simulink model "ASDdc_Governor"  (R2016b)
settings: configuration reference "CodeGenConfigSet" (kept outside this file)
values from neighbouring files (symbols this model uses):
  ASDdc_trqLimMax_C = Calibration.Parameter    [init_ASDdc_Governor.m]    (also in init_ASDdc_Governor_SIL.m = Simulink.Parameter)
  ASDdc_trqLimMin_C = Calibration.Parameter    [init_ASDdc_Governor.m]    (also in init_ASDdc_Governor_SIL.m = Simulink.Parameter)
  ASDdc_vLimIni_C = Calibration.Parameter    [init_ASDdc_Governor.m]    (also in init_ASDdc_Governor_SIL.m = Simulink.Parameter)
  PthSet_trqASDdcInit_C = Calibration.Parameter    [init_ASDdc_Governor.m]    (also in init_ASDdc_Governor_SIL.m = Simulink.Parameter)
undefined symbols (not defined in the file or in its folder): ASDdc_Governor_DT, EngState_conv
libraries: CXLib x3
settings Model: Creator=lenovo  LastModifiedBy=lenovo
settings ConfigSetRef: SourceLocation=Base Workspace

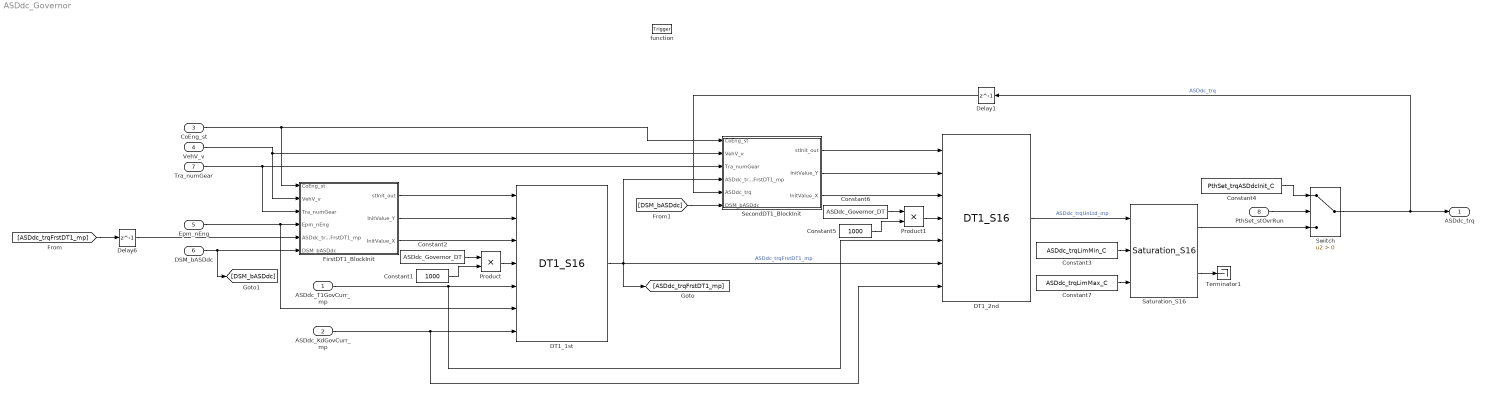
== system ASDdc_Governor ==
  ASDdc_T1GovCurr_mp : Inport  Tag=ms  Description=Current parameter T1 for ASD disturbance compensator  OutMin=0  OutMax=65535  OutDataTypeStr=RailDT1_ms
  ASDdc_KdGovCurr_mp : Inport  Description=Current parameter Kd for ASD disturbance compensator  Port=2  OutMin=0  OutMax=15  OutDataTypeStr=Pid_Kp_Kd
  CoEng_st : Inport  Description=Engine coordinator state  Port=3  OutDataTypeStr=Enum: EngState_conv
  VehV_v : Inport  Tag=km/h  Description=Vehicle speed  Port=4  OutMin=0  OutMax=250  OutDataTypeStr=VehSpeed_km_h
  Epm_nEng : Inport  Tag=rpm  Description=Engine speed  Port=5  OutMin=0  OutMax=6000  OutDataTypeStr=EngSpeed_rpm
  DSM_bASDdc : Inport  Description=state of Fid_ASDDc  Port=6  OutMin=0  OutMax=1  OutDataTypeStr=boolean
  Tra_numGear : Inport  Description=Current gear information  Port=7  OutMin=-128  OutMax=127  OutDataTypeStr=Tra_num
  PthSet_stOvrRun : Inport  Description=State of overrun detection (0: No overrun; 1: overrun)  Port=8  OutMin=0  OutMax=1  OutDataTypeStr=boolean
  function : TriggerPort  TriggerType=function-call  VariantControl=Variant
  Constant1 : Constant  RequirementInfo={'other' 'APP_requirements.doc' '@Simulink_requirement_item_25' 'true' '手动开关' '' } %GIDa_e3d2db55_e091_4804_b405_e3bf1d89a990  Value=1000  OutDataTypeStr=uint32
  Constant2 : Constant  RequirementInfo={'other' 'APP_requirements.doc' '@Simulink_requirement_item_25' 'true' '手动开关' '' } %GIDa_d3ebbc02_8a2a_474e_954c_97ec141fe6cb  Value=ASDdc_Governor_DT
  Constant3 : Constant  RequirementInfo={'other' 'APP_requirements.doc' '@Simulink_requirement_item_25' 'true' '手动开关' '' } %GIDa_af684717_0e96_4c26_8bce_fac0e3667dc0  Value=ASDdc_trqLimMin_C  SampleTime=-1
  Constant4 : Constant  RequirementInfo={'other' 'APP_requirements.doc' '@Simulink_requirement_item_25' 'true' '手动开关' '' } %GIDa_d8318f6c_a07c_4d1c_adda_9fb670b3e1e3  Value=PthSet_trqASDdcInit_C  SampleTime=-1
  Constant5 : Constant  RequirementInfo={'other' 'APP_requirements.doc' '@Simulink_requirement_item_25' 'true' '手动开关' '' } %GIDa_6b95edb5_017f_4d36_805f_c1c3801a481a  Value=1000  OutDataTypeStr=uint32
  Constant6 : Constant  RequirementInfo={'other' 'APP_requirements.doc' '@Simulink_requirement_item_25' 'true' '手动开关' '' } %GIDa_682dba5f_241e_4249_aa6e_798392b0670d  Value=ASDdc_Governor_DT
  Constant7 : Constant  RequirementInfo={'other' 'APP_requirements.doc' '@Simulink_requirement_item_25' 'true' '手动开关' '' } %GIDa_b9d68d89_a686_4446_af65_722001efe125  Value=ASDdc_trqLimMax_C  SampleTime=-1
  DT1_1st : CXLib/DT1_S16
  DT1_2nd : CXLib/DT1_S16
  Delay1 : Delay  DelayLength=1  InitialCondition=0
  Delay6 : Delay  DelayLength=1  InitialCondition=0
  FirstDT1_BlockInit : Subsystem
  Product : Product  OutDataTypeStr=Inherit: Inherit via back propagation
  Product1 : Product  OutDataTypeStr=Inherit: Inherit via back propagation
  Saturation_S16 : CXLib/Saturation_S16
  SecondDT1_BlockInit : Subsystem
  Switch : Switch  Criteria=u2 > Threshold
  Terminator1 : Terminator
  ASDdc_trq : Outport  Tag=Nm  Description=ASD disturbance compensator torque output  OutMin=-3000  OutMax=3000  OutDataTypeStr=Trq_Nm
  wires:
  Delay1/1 -> SecondDT1_BlockInit/5(ASDdc_trq)
  Delay6/1 -> FirstDT1_BlockInit/5(ASDdc_trqFrstDT1_mp)
  [ASDdc_trqFrstDT1_mp] -> Delay6/1
  Tra_numGear/1 -> FirstDT1_BlockInit/3(Tra_numGear), SecondDT1_BlockInit/3(Tra_numGear)
  Epm_nEng/1 -> DT1_1st/6, FirstDT1_BlockInit/4(Epm_nEng)
  SecondDT1_BlockInit/1(stInit_out) -> DT1_2nd/1
  SecondDT1_BlockInit/2(InitValue_Y) -> DT1_2nd/2
  SecondDT1_BlockInit/3(InitValue_X) -> DT1_2nd/3
  FirstDT1_BlockInit/1(stInit_out) -> DT1_1st/1
  FirstDT1_BlockInit/2(InitValue_Y) -> DT1_1st/2
  FirstDT1_BlockInit/3(InitValue_X) -> DT1_1st/3
  ASDdc_KdGovCurr_mp/1 -> DT1_2nd/7, DT1_1st/7
  ASDdc_T1GovCurr_mp/1 -> DT1_2nd/5, DT1_1st/5
  VehV_v/1 -> FirstDT1_BlockInit/2(VehV_v), SecondDT1_BlockInit/2(VehV_v)
  CoEng_st/1 -> FirstDT1_BlockInit/1(CoEng_st), SecondDT1_BlockInit/1(CoEng_st)
  Switch/1 -> ASDdc_trq/1, Delay1/1  "ASDdc_trq"
  Saturation_S16/2 -> Terminator1/1
  Constant7/1 -> Saturation_S16/3
  Constant3/1 -> Saturation_S16/2
  DT1_2nd/1 -> Saturation_S16/1  "ASDdc_trqUnLtd_mp"
  DT1_1st/1 -> SecondDT1_BlockInit/4(ASDdc_trqFrstDT1_mp), DT1_2nd/6, [ASDdc_trqFrstDT1_mp]  "ASDdc_trqFrstDT1_mp"
  DSM_bASDdc/1 -> FirstDT1_BlockInit/6(DSM_bASDdc), [DSM_bASDdc]
  [DSM_bASDdc] -> SecondDT1_BlockInit/6(DSM_bASDdc)
  Product/1 -> DT1_1st/4
  Constant2/1 -> Product/1
  Constant1/1 -> Product/2
  Constant6/1 -> Product1/1
  Constant5/1 -> Product1/2
  Product1/1 -> DT1_2nd/4
  PthSet_stOvrRun/1 -> Switch/2
  Saturation_S16/1 -> Switch/3
  Constant4/1 -> Switch/1

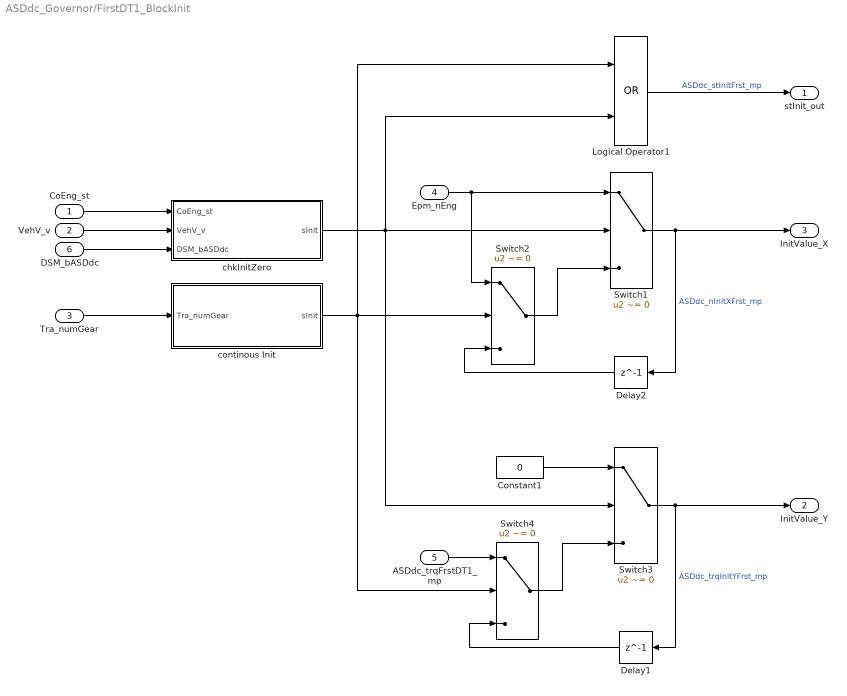
== system ASDdc_Governor/FirstDT1_BlockInit ==
  CoEng_st : Inport
  VehV_v : Inport  Port=2
  Tra_numGear : Inport  Port=3
  Epm_nEng : Inport  Port=4
  ASDdc_trqFrstDT1_mp : Inport  Port=5
  DSM_bASDdc : Inport  Description=state of Fid_ASDDc  Port=6
  Constant1 : Constant  RequirementInfo={'other' 'APP_requirements.doc' '@Simulink_requirement_item_25' 'true' '手动开关' '' } %GIDa_41ce0f65_227c_46f1_80d2_1d565a574450  Value=0  OutDataTypeStr=Inherit: Inherit via back propagation
  Delay1 : Delay  DelayLength=1  InitialCondition=0
  Delay2 : Delay  DelayLength=1  InitialCondition=0
  Logical Operator1 : Logic  Operator=OR  OutDataTypeStr=boolean
  Switch{1..4} (4 alike) : Switch  Criteria=u2 ~= 0  SaturateOnIntegerOverflow=on  InputSameDT=on
  chkInitZero : Subsystem
  continous Init : Subsystem
  stInit_out : Outport
  InitValue_Y : Outport  Port=2
  InitValue_X : Outport  Port=3
  wires:
  Tra_numGear/1 -> continous Init/1(Tra_numGear)
  VehV_v/1 -> chkInitZero/2(VehV_v)
  CoEng_st/1 -> chkInitZero/1(CoEng_st)
  ASDdc_trqFrstDT1_mp/1 -> Switch4/1
  Epm_nEng/1 -> Switch1/1, Switch2/1
  continous Init/1(sInit) -> Logical Operator1/1, Switch2/2, Switch4/2
  Switch3/1 -> Delay1/1, InitValue_Y/1  "ASDdc_trqInitYFrst_mp"
  Constant1/1 -> Switch3/1
  chkInitZero/1(sInit) -> Logical Operator1/2, Switch1/2, Switch3/2
  Switch4/1 -> Switch3/3
  Delay1/1 -> Switch4/3
  Logical Operator1/1 -> stInit_out/1  "ASDdc_stInitFrst_mp"
  Switch2/1 -> Switch1/3
  Switch1/1 -> Delay2/1, InitValue_X/1  "ASDdc_nInitXFrst_mp"
  Delay2/1 -> Switch2/3
  DSM_bASDdc/1 -> chkInitZero/3(DSM_bASDdc)

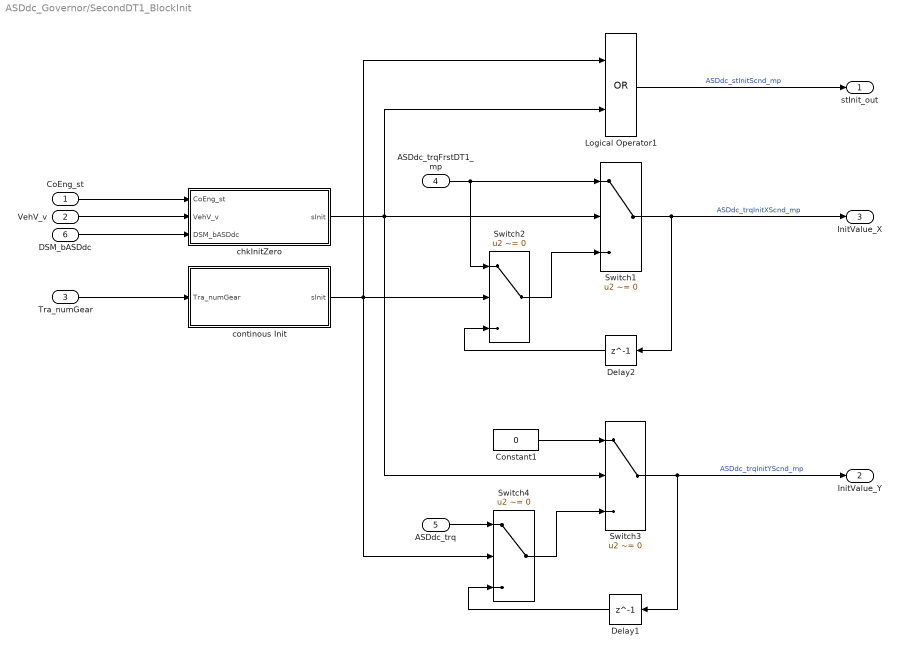
== system ASDdc_Governor/SecondDT1_BlockInit ==
  CoEng_st : Inport
  VehV_v : Inport  Port=2
  Tra_numGear : Inport  Port=3
  ASDdc_trqFrstDT1_mp : Inport  Port=4
  ASDdc_trq : Inport  Port=5
  DSM_bASDdc : Inport  Description=state of Fid_ASDDc  Port=6
  Constant1 : Constant  RequirementInfo={'other' 'APP_requirements.doc' '@Simulink_requirement_item_25' 'true' '手动开关' '' } %GIDa_41ce0f65_227c_46f1_80d2_1d565a574450  Value=0  OutDataTypeStr=Inherit: Inherit via back propagation
  Delay1 : Delay  DelayLength=1  InitialCondition=0
  Delay2 : Delay  DelayLength=1  InitialCondition=0
  Logical Operator1 : Logic  Operator=OR  OutDataTypeStr=boolean
  Switch{1..4} (4 alike) : Switch  Criteria=u2 ~= 0  SaturateOnIntegerOverflow=on  InputSameDT=on
  chkInitZero : Subsystem
  continous Init : Subsystem
  stInit_out : Outport
  InitValue_Y : Outport  Port=2
  InitValue_X : Outport  Port=3
  wires:
  Tra_numGear/1 -> continous Init/1(Tra_numGear)
  VehV_v/1 -> chkInitZero/2(VehV_v)
  CoEng_st/1 -> chkInitZero/1(CoEng_st)
  Delay2/1 -> Switch2/3
  Switch1/1 -> Delay2/1, InitValue_X/1  "ASDdc_trqInitXScnd_mp"
  Switch2/1 -> Switch1/3
  Logical Operator1/1 -> stInit_out/1  "ASDdc_stInitScnd_mp"
  Delay1/1 -> Switch4/3
  Switch4/1 -> Switch3/3
  chkInitZero/1(sInit) -> Logical Operator1/2, Switch3/2, Switch1/2
  Constant1/1 -> Switch3/1
  Switch3/1 -> Delay1/1, InitValue_Y/1  "ASDdc_trqInitYScnd_mp"
  continous Init/1(sInit) -> Switch4/2, Switch2/2, Logical Operator1/1
  ASDdc_trqFrstDT1_mp/1 -> Switch2/1, Switch1/1
  ASDdc_trq/1 -> Switch4/1
  DSM_bASDdc/1 -> chkInitZero/3(DSM_bASDdc)

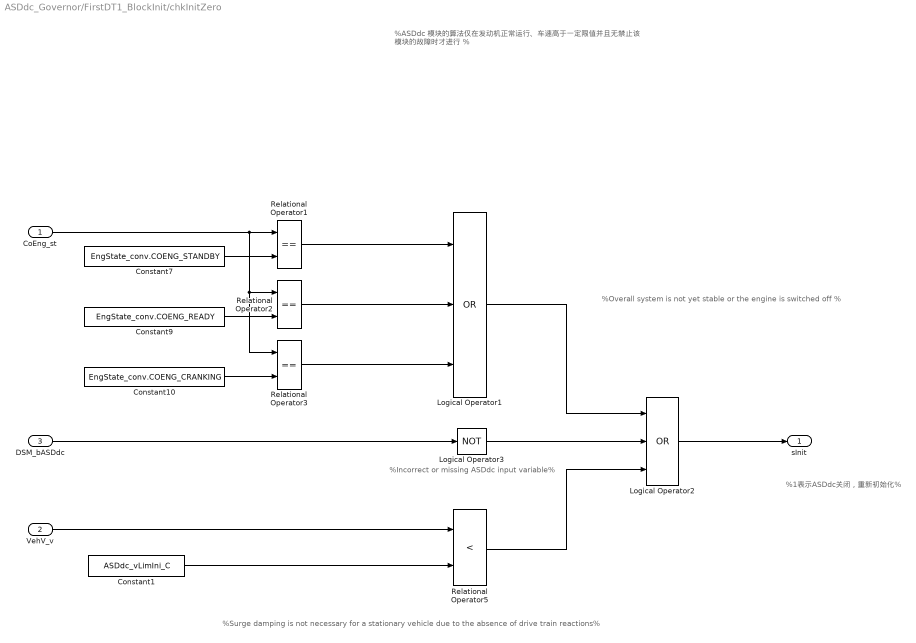
== system ASDdc_Governor/FirstDT1_BlockInit/chkInitZero ==
  note: %ASDdc 模块的算法仅在发动机正常运行、车速高于一定限值并且无禁止该
      | 模块的故障时才进行 %
  note: %1表示ASDdc关闭，重新初始化%
  note: %Overall system is not yet stable or the engine is switched off %
  note: %Incorrect or missing ASDdc input variable%
  note: %Surge damping is not necessary for a stationary vehicle due to the absence of drive train reactions%
  CoEng_st : Inport
  VehV_v : Inport  Port=2
  DSM_bASDdc : Inport  Description=state of Fid_ASDDc  Port=3
  Constant1 : Constant  RequirementInfo={'other' 'APP_requirements.doc' '@Simulink_requirement_item_25' 'true' '手动开关' '' } %GIDa_c1cc4cd8_0d9b_48ec_a78d_d033a54bf682  Value=ASDdc_vLimIni_C  SampleTime=-1
  Constant10 : Constant  RequirementInfo={'other' 'APP_requirements.doc' '@Simulink_requirement_item_25' 'true' '手动开关' '' } %GIDa_210c9743_263f_42ed_9164_536893c43ee7  Value=EngState_conv.COENG_CRANKING  OutDataTypeStr=Inherit: Inherit via back propagation  SampleTime=-1
  Constant7 : Constant  RequirementInfo={'other' 'APP_requirements.doc' '@Simulink_requirement_item_25' 'true' '手动开关' '' } %GIDa_104c9b9c_13d9_43c4_8c84_72634ccd6a8a  Value=EngState_conv.COENG_STANDBY  OutDataTypeStr=Inherit: Inherit via back propagation  SampleTime=-1
  Constant9 : Constant  RequirementInfo={'other' 'APP_requirements.doc' '@Simulink_requirement_item_25' 'true' '手动开关' '' } %GIDa_202de214_395d_47e8_aba5_15a49444dd5d  Value=EngState_conv.COENG_READY  OutDataTypeStr=Inherit: Inherit via back propagation  SampleTime=-1
  Logical Operator1 : Logic  Operator=OR  Inputs=3  OutDataTypeStr=boolean
  Logical Operator2 : Logic  Operator=OR  Inputs=3  OutDataTypeStr=boolean
  Logical Operator3 : Logic  Operator=NOT  Inputs=3  OutDataTypeStr=boolean
  Relational Operator1 : RelationalOperator  Operator===  OutDataTypeStr=boolean  RndMeth=Simplest  InputSameDT=on
  Relational Operator2 : RelationalOperator  Operator===  OutDataTypeStr=boolean  RndMeth=Simplest  InputSameDT=on
  Relational Operator3 : RelationalOperator  Operator===  OutDataTypeStr=boolean  RndMeth=Simplest  InputSameDT=on
  Relational Operator5 : RelationalOperator  Operator=<  OutDataTypeStr=boolean  RndMeth=Simplest  InputSameDT=on
  sInit : Outport
  wires:
  Constant1/1 -> Relational Operator5/2
  Logical Operator1/1 -> Logical Operator2/1
  Constant9/1 -> Relational Operator2/2
  Relational Operator2/1 -> Logical Operator1/2
  Constant10/1 -> Relational Operator3/2
  Relational Operator5/1 -> Logical Operator2/3
  Relational Operator3/1 -> Logical Operator1/3
  Relational Operator1/1 -> Logical Operator1/1
  VehV_v/1 -> Relational Operator5/1
  Logical Operator2/1 -> sInit/1
  DSM_bASDdc/1 -> Logical Operator3/1
  CoEng_st/1 -> Relational Operator3/1, Relational Operator2/1, Relational Operator1/1
  Constant7/1 -> Relational Operator1/2
  Logical Operator3/1 -> Logical Operator2/2

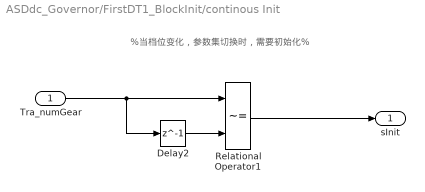
== system ASDdc_Governor/FirstDT1_BlockInit/continous Init ==
  note: %当档位变化，参数集切换时，需要初始化%
  Tra_numGear : Inport
  Delay2 : Delay  DelayLength=1  InitialCondition=0
  Relational Operator1 : RelationalOperator  Operator=~=  OutDataTypeStr=boolean  RndMeth=Simplest  InputSameDT=on
  sInit : Outport
  wires:
  Relational Operator1/1 -> sInit/1
  Tra_numGear/1 -> Relational Operator1/1, Delay2/1
  Delay2/1 -> Relational Operator1/2

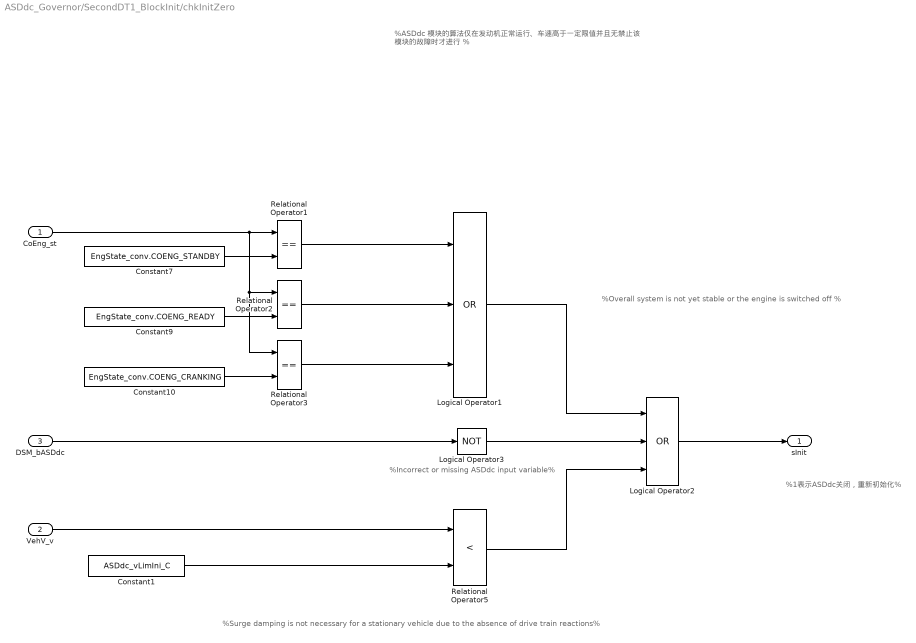
== system ASDdc_Governor/SecondDT1_BlockInit/chkInitZero ==
  note: %Surge damping is not necessary for a stationary vehicle due to the absence of drive train reactions%
  note: %Incorrect or missing ASDdc input variable%
  note: %Overall system is not yet stable or the engine is switched off %
  note: %1表示ASDdc关闭，重新初始化%
  note: %ASDdc 模块的算法仅在发动机正常运行、车速高于一定限值并且无禁止该
      | 模块的故障时才进行 %
  CoEng_st : Inport
  VehV_v : Inport  Port=2
  DSM_bASDdc : Inport  Description=state of Fid_ASDDc  Port=3
  Constant1 : Constant  RequirementInfo={'other' 'APP_requirements.doc' '@Simulink_requirement_item_25' 'true' '手动开关' '' } %GIDa_c1cc4cd8_0d9b_48ec_a78d_d033a54bf682  Value=ASDdc_vLimIni_C  SampleTime=-1
  Constant10 : Constant  RequirementInfo={'other' 'APP_requirements.doc' '@Simulink_requirement_item_25' 'true' '手动开关' '' } %GIDa_210c9743_263f_42ed_9164_536893c43ee7  Value=EngState_conv.COENG_CRANKING  OutDataTypeStr=Inherit: Inherit via back propagation  SampleTime=-1
  Constant7 : Constant  RequirementInfo={'other' 'APP_requirements.doc' '@Simulink_requirement_item_25' 'true' '手动开关' '' } %GIDa_104c9b9c_13d9_43c4_8c84_72634ccd6a8a  Value=EngState_conv.COENG_STANDBY  OutDataTypeStr=Inherit: Inherit via back propagation  SampleTime=-1
  Constant9 : Constant  RequirementInfo={'other' 'APP_requirements.doc' '@Simulink_requirement_item_25' 'true' '手动开关' '' } %GIDa_202de214_395d_47e8_aba5_15a49444dd5d  Value=EngState_conv.COENG_READY  OutDataTypeStr=Inherit: Inherit via back propagation  SampleTime=-1
  Logical Operator1 : Logic  Operator=OR  Inputs=3  OutDataTypeStr=boolean
  Logical Operator2 : Logic  Operator=OR  Inputs=3  OutDataTypeStr=boolean
  Logical Operator3 : Logic  Operator=NOT  Inputs=3  OutDataTypeStr=boolean
  Relational Operator1 : RelationalOperator  Operator===  OutDataTypeStr=boolean  RndMeth=Simplest  InputSameDT=on
  Relational Operator2 : RelationalOperator  Operator===  OutDataTypeStr=boolean  RndMeth=Simplest  InputSameDT=on
  Relational Operator3 : RelationalOperator  Operator===  OutDataTypeStr=boolean  RndMeth=Simplest  InputSameDT=on
  Relational Operator5 : RelationalOperator  Operator=<  OutDataTypeStr=boolean  RndMeth=Simplest  InputSameDT=on
  sInit : Outport
  wires:
  Logical Operator3/1 -> Logical Operator2/2
  Constant7/1 -> Relational Operator1/2
  CoEng_st/1 -> Relational Operator1/1, Relational Operator2/1, Relational Operator3/1
  DSM_bASDdc/1 -> Logical Operator3/1
  Logical Operator2/1 -> sInit/1
  VehV_v/1 -> Relational Operator5/1
  Relational Operator1/1 -> Logical Operator1/1
  Relational Operator3/1 -> Logical Operator1/3
  Relational Operator5/1 -> Logical Operator2/3
  Constant10/1 -> Relational Operator3/2
  Relational Operator2/1 -> Logical Operator1/2
  Constant9/1 -> Relational Operator2/2
  Logical Operator1/1 -> Logical Operator2/1
  Constant1/1 -> Relational Operator5/2

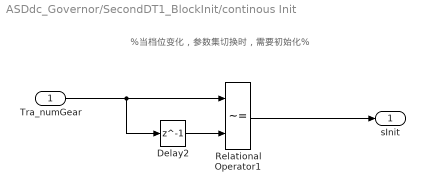
== system ASDdc_Governor/SecondDT1_BlockInit/continous Init ==
  note: %当档位变化，参数集切换时，需要初始化%
  Tra_numGear : Inport
  Delay2 : Delay  DelayLength=1  InitialCondition=0
  Relational Operator1 : RelationalOperator  Operator=~=  OutDataTypeStr=boolean  RndMeth=Simplest  InputSameDT=on
  sInit : Outport
  wires:
  Delay2/1 -> Relational Operator1/2
  Tra_numGear/1 -> Delay2/1, Relational Operator1/1
  Relational Operator1/1 -> sInit/1
